simulink model "DynamicEquation3"  (R2017b)
settings: configuration reference "cs" (kept outside this file)
undefined symbols (not defined in the file or in its folder): Configuration, Sim_Control
settings Model: Creator=One  LastModifiedBy=One
settings ConfigSetRef: SourceLocation=Base Workspace

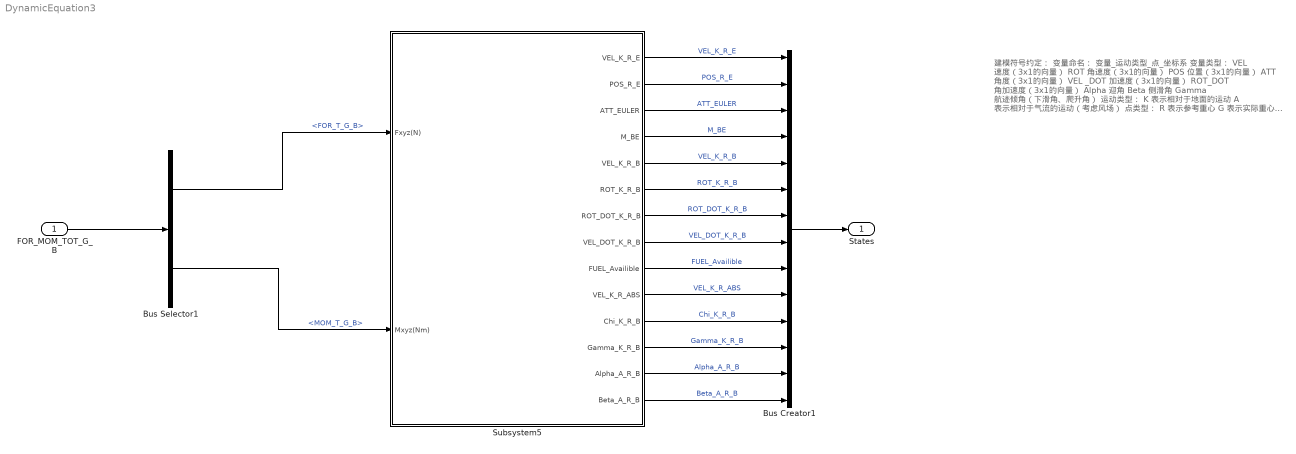
== system DynamicEquation3 ==
  note: 建模符号约定：
      | 变量命名：
      | 变量_运动类型_点_坐标系
      |
      | 变量类型：
      | VEL 速度（3x1的向量）
      | ROT 角速度（3x1的向量）
      | POS 位置（3x1的向量）
      | ATT 角度（3x1的向量）
      | VEL _DOT 加速度（3x1的向量）
      | ROT_DOT 角加速度（3x1的向量）
      | Alpha 迎角
      | Beta 侧滑角
      | Gamma 航迹倾角（下滑角、爬升角）
      | 运动类型：
      | K 表示相对于地面的运动
      | A 表示相对于气流的运动（考虑风场）
      | 点类型：
      | R 表示参考重心
      | G 表示实际重心
      | 坐标系类型：
      | B 机体系
      | E 地面系 ABS 与坐标系无关，表示该变量的绝对值
  FOR_MOM_TOT_G_B : Inport  OutDataTypeStr=Bus: FOR_MOM_TOT_BUS
  Bus Creator1 : BusCreator  Inputs=14  OutDataTypeStr=Bus: States_BUS
  Bus Selector1 : BusSelector  OutputSignals=FOR_T_G_B,MOM_T_G_B
  Subsystem5 : Subsystem
  States : Outport  OutDataTypeStr=Bus: States_BUS
  wires:
  Bus Selector1/1 -> Subsystem5/1(Fxyz(N))  "<FOR_T_G_B>"
  FOR_MOM_TOT_G_B/1 -> Bus Selector1/1
  Bus Selector1/2 -> Subsystem5/2(Mxyz(Nm))  "<MOM_T_G_B>"
  Subsystem5/1(VEL_K_R_E) -> Bus Creator1/1  "VEL_K_R_E"
  Subsystem5/2(POS_R_E) -> Bus Creator1/2  "POS_R_E"
  Subsystem5/3(ATT_EULER) -> Bus Creator1/3  "ATT_EULER"
  Subsystem5/4(M_BE) -> Bus Creator1/4  "M_BE"
  Subsystem5/5(VEL_K_R_B) -> Bus Creator1/5  "VEL_K_R_B"
  Subsystem5/6(ROT_K_R_B) -> Bus Creator1/6  "ROT_K_R_B"
  Subsystem5/7(ROT_DOT_K_R_B) -> Bus Creator1/7  "ROT_DOT_K_R_B"
  Subsystem5/8(VEL_DOT_K_R_B) -> Bus Creator1/8  "VEL_DOT_K_R_B"
  Subsystem5/9(FUEL_Availible) -> Bus Creator1/9  "FUEL_Availible"
  Subsystem5/10(VEL_K_R_ABS) -> Bus Creator1/10  "VEL_K_R_ABS"
  Subsystem5/11(Chi_K_R_B) -> Bus Creator1/11  "Chi_K_R_B"
  Subsystem5/12(Gamma_K_R_B) -> Bus Creator1/12  "Gamma_K_R_B"
  Subsystem5/13(Alpha_A_R_B) -> Bus Creator1/13  "Alpha_A_R_B"
  Subsystem5/14(Beta_A_R_B) -> Bus Creator1/14  "Beta_A_R_B"
  Bus Creator1/1 -> States/1

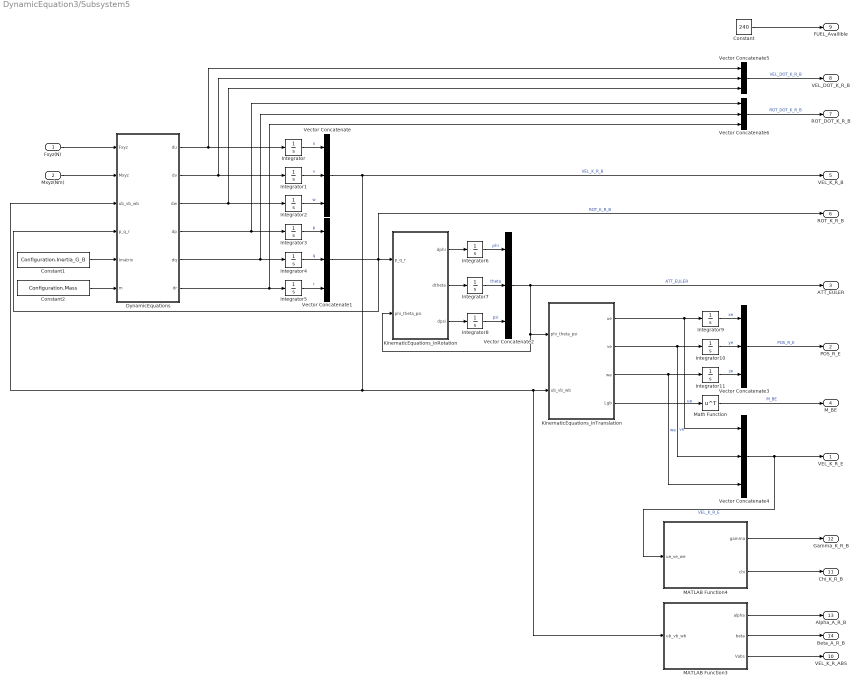
== system DynamicEquation3/Subsystem5 ==
  Fxyz(N) : Inport
  Mxyz(Nm) : Inport  Port=2
  Constant : Constant  Value=240
  Constant1 : Constant  Value=Configuration.Inertia_G_B
  Constant2 : Constant  Value=Configuration.Mass
  DynamicEquations : MATLAB Function  TreatAsAtomicUnit=on
  Integrator : Integrator  InitialCondition=Sim_Control.init(2,1)  ContinuousStateAttributes='ub'
  Integrator1 : Integrator  InitialCondition=Sim_Control.init(2,2)  ContinuousStateAttributes='vb'
  Integrator10 : Integrator  InitialCondition=Sim_Control.init(1,2)  ContinuousStateAttributes='ye'
  Integrator11 : Integrator  InitialCondition=Sim_Control.init(1,3)  ContinuousStateAttributes='ze'
  Integrator2 : Integrator  InitialCondition=Sim_Control.init(2,3)  ContinuousStateAttributes='wb'
  Integrator3 : Integrator  InitialCondition=Sim_Control.init(4,1)  ContinuousStateAttributes='p'
  Integrator4 : Integrator  InitialCondition=Sim_Control.init(4,2)  ContinuousStateAttributes='q'
  Integrator5 : Integrator  InitialCondition=Sim_Control.init(4,3)  ContinuousStateAttributes='r'
  Integrator6 : Integrator  InitialCondition=Sim_Control.init(3,1)  ContinuousStateAttributes='phi'
  Integrator7 : Integrator  InitialCondition=Sim_Control.init(3,2)  ContinuousStateAttributes='theta'
  Integrator8 : Integrator  InitialCondition=Sim_Control.init(3,3)  ContinuousStateAttributes='psi'
  Integrator9 : Integrator  InitialCondition=Sim_Control.init(1,1)  ContinuousStateAttributes='xe'
  KinematicEquations_InRotation : MATLAB Function  TreatAsAtomicUnit=on
  KinematicEquations_InTranslation : MATLAB Function  TreatAsAtomicUnit=on
  MATLAB Function3 : MATLAB Function  TreatAsAtomicUnit=on
  MATLAB Function4 : MATLAB Function  TreatAsAtomicUnit=on
  Math Function : Math  Operator=transpose  SaturateOnIntegerOverflow=on
  Vector Concatenate{,1..6} (7 alike) : Concatenate  NumInputs=3
  VEL_K_R_E : Outport
  POS_R_E : Outport  Port=2
  ATT_EULER : Outport  Port=3
  M_BE : Outport  Port=4
  VEL_K_R_B : Outport  Port=5
  ROT_K_R_B : Outport  Port=6
  ROT_DOT_K_R_B : Outport  Port=7
  VEL_DOT_K_R_B : Outport  Port=8
  FUEL_Availible : Outport  Port=9
  VEL_K_R_ABS : Outport  Port=10
  Chi_K_R_B : Outport  Port=11
  Gamma_K_R_B : Outport  Port=12
  Alpha_A_R_B : Outport  Port=13
  Beta_A_R_B : Outport  Port=14
  wires:
  DynamicEquations/5(dq) -> Vector Concatenate6/2, Integrator4/1
  Integrator2/1 -> Vector Concatenate/3  "w"
  Integrator/1 -> Vector Concatenate/1  "u"
  DynamicEquations/3(dw) -> Vector Concatenate5/3, Integrator2/1
  KinematicEquations_InRotation/3(dpsi) -> Integrator8/1
  KinematicEquations_InRotation/2(dtheta) -> Integrator7/1
  Vector Concatenate2/1 -> ATT_EULER/1, KinematicEquations_InRotation/2(phi_theta_psi), KinematicEquations_InTranslation/1(phi_theta_psi)  "ATT_EULER"
  Vector Concatenate/1 -> VEL_K_R_B/1, DynamicEquations/3(ub_vb_wb), KinematicEquations_InTranslation/2(ub_vb_wb), MATLAB Function3/1(ub_vb_wb)  "VEL_K_R_B"
  KinematicEquations_InTranslation/1(ue) -> Vector Concatenate4/1, Integrator9/1  "ue"
  KinematicEquations_InTranslation/3(we) -> Vector Concatenate4/3, Integrator11/1  "we"
  DynamicEquations/2(dv) -> Vector Concatenate5/2, Integrator1/1
  Integrator4/1 -> Vector Concatenate1/2  "q"
  Integrator5/1 -> Vector Concatenate1/3  "r"
  Integrator3/1 -> Vector Concatenate1/1  "p"
  KinematicEquations_InRotation/1(dphi) -> Integrator6/1
  DynamicEquations/1(du) -> Vector Concatenate5/1, Integrator/1
  Integrator1/1 -> Vector Concatenate/2  "v"
  DynamicEquations/6(dr) -> Vector Concatenate6/3, Integrator5/1
  Integrator8/1 -> Vector Concatenate2/3  "psi"
  Integrator6/1 -> Vector Concatenate2/1  "phi"
  Vector Concatenate1/1 -> DynamicEquations/4(p_q_r), ROT_K_R_B/1, KinematicEquations_InRotation/1(p_q_r)  "ROT_K_R_B"
  Integrator7/1 -> Vector Concatenate2/2  "theta"
  Integrator11/1 -> Vector Concatenate3/3  "ze"
  DynamicEquations/4(dp) -> Vector Concatenate6/1, Integrator3/1
  Integrator9/1 -> Vector Concatenate3/1  "xe"
  KinematicEquations_InTranslation/2(ve) -> Vector Concatenate4/2, Integrator10/1  "ve"
  Integrator10/1 -> Vector Concatenate3/2  "ye"
  Fxyz(N)/1 -> DynamicEquations/1(Fxyz)
  Mxyz(Nm)/1 -> DynamicEquations/2(Mxyz)
  Vector Concatenate3/1 -> POS_R_E/1  "POS_R_E"
  Vector Concatenate4/1 -> VEL_K_R_E/1, MATLAB Function4/1(ue_ve_we)  "VEL_K_R_E"
  KinematicEquations_InTranslation/4(Lgb) -> Math Function/1
  Math Function/1 -> M_BE/1  "M_BE"
  Vector Concatenate6/1 -> ROT_DOT_K_R_B/1  "ROT_DOT_K_R_B"
  Vector Concatenate5/1 -> VEL_DOT_K_R_B/1  "VEL_DOT_K_R_B"
  Constant/1 -> FUEL_Availible/1
  MATLAB Function3/1(alpha) -> Alpha_A_R_B/1
  MATLAB Function3/2(beta) -> Beta_A_R_B/1
  MATLAB Function3/3(Vabs) -> VEL_K_R_ABS/1
  MATLAB Function4/1(gamma) -> Gamma_K_R_B/1
  MATLAB Function4/2(chi) -> Chi_K_R_B/1
  Constant1/1 -> DynamicEquations/5(Imatrix)
  Constant2/1 -> DynamicEquations/6(m)

== matlab function DynamicEquation3/Subsystem5/KinematicEquations_InRotation ==
  data: p_q_r input; dphi output; phi_theta_psi input; dtheta output; dpsi output
function [dphi, dtheta, dpsi] = fcn(p_q_r, phi_theta_psi)
p = p_q_r(1);
q = p_q_r(2);
r = p_q_r(3);
phi = phi_theta_psi(1);
theta = phi_theta_psi(2);

dphi = p+tan(theta)*(q*sin(phi)+r*cos(phi));
dtheta = q*cos(phi)-r*sin(phi);
dpsi = (q*sin(phi)+r*cos(phi))/cos(theta);

end

== matlab function DynamicEquation3/Subsystem5/DynamicEquations ==
  data: Fxyz input; du output; Mxyz input; ub_vb_wb input; p_q_r input; Imatrix input; m input; dv output; dw output; dp output; dq output; dr output
function [du, dv, dw, dp, dq, dr] = fcn(Fxyz, Mxyz, ub_vb_wb, p_q_r, Imatrix, m)
Fx = Fxyz(1);
Fy = Fxyz(2);
Fz = Fxyz(3);
Mx = Mxyz(1);
My = Mxyz(2);
Mz = Mxyz(3);
u = ub_vb_wb(1);
v = ub_vb_wb(2);
w = ub_vb_wb(3);
p = p_q_r(1);
q = p_q_r(2);
r = p_q_r(3);
Ix = Imatrix(1,1);
Iy = Imatrix(2,2);
Iz = Imatrix(3,3);
Izx = Imatrix(1,3);

du=-w*q+v*r+Fx/m;
dv=-u*r+w*p+Fy/m;
dw=-v*p+u*q+Fz/m;
dp=(-(Izx*Izx+Iz*Iz-Iz*Iy)*q*r+Izx*(Iz-Iy+Ix)*p*q+Izx*Mz+Iz*Mx)/(Ix*Iz-Izx*Izx);
dq=(-Izx*(p*p-r*r)-(Ix-Iz)*r*p+My)/(Iy);
dr=(-Izx*(Ix+Iz-Iy)*q*r+(-Ix*Iy+Ix*Ix+Izx*Izx)*p*q+Ix*Mz+Izx*Mx)/(Ix*Iz-Izx*Izx);
end

== matlab function DynamicEquation3/Subsystem5/KinematicEquations_InTranslation ==
  data: phi_theta_psi input; ub_vb_wb input; ue output; ve output; we output; Lgb output
function [ue, ve, we, Lgb] = fcn(phi_theta_psi, ub_vb_wb)
phi = phi_theta_psi(1);
theta = phi_theta_psi(2);
psi = phi_theta_psi(3);
% u = ub_vb_wb(1);
% v = ub_vb_wb(2);
% w = ub_vb_wb(3);

Lgb=...
  [ cos(psi)*cos(theta), cos(psi)*sin(phi)*sin(theta) - cos(phi)*sin(psi), sin(phi)*sin(psi) + cos(phi)*cos(psi)*sin(theta);
    cos(theta)*sin(psi), cos(phi)*cos(psi) + sin(phi)*sin(psi)*sin(theta), cos(phi)*sin(psi)*sin(theta) - cos(psi)*sin(phi);
          -sin(theta),                        cos(theta)*sin(phi),                        cos(phi)*cos(theta)];
 
ue_ve_we=Lgb*ub_vb_wb;
ue = ue_ve_we(1);
ve = ue_ve_we(2);
we = ue_ve_we(3);
end

== matlab function DynamicEquation3/Subsystem5/MATLAB Function4 ==
  data: ue_ve_we input; gamma output; chi output
function [gamma, chi] = fcn(ue_ve_we)
u = ue_ve_we(1);
v = ue_ve_we(2);
w = ue_ve_we(3);

Vabs = sqrt(u*u+v*v+w*w);
if Vabs<0.01
    Vabs = 0.01;
end
gamma = asin(w/Vabs);
chi = atan(v/u);
if chi<0
    chi = chi+2*pi;
end


end

== matlab function DynamicEquation3/Subsystem5/MATLAB Function3 ==
  data: ub_vb_wb input; alpha output; beta output; Vabs output
function [alpha, beta, Vabs] = fcn(ub_vb_wb)
u = ub_vb_wb(1);
v = ub_vb_wb(2);
w = ub_vb_wb(3);

alpha = atan(w/u);
Vabs = sqrt(u*u+v*v+w*w);
if Vabs<0.01
    Vabs = 0.01;
end
beta = asin(v/Vabs);

end
